simulink model "Fig221"  (R2014b)
settings: Solver=ode3  StartTime=0.0  StopTime=10.007  FixedStep=2e-5  RelTol=1e-5
undefined symbols (not defined in the file): gcbh, rcfiltgaincompat
libraries: commchan3 x1, commsink2 x1, dsparch4 x1, dspsigops x1, commrandsrc2 x1, commfilt2 x1
settings Model: Creator=Dennis Silage  LastModifiedBy=Silage
settings DataIOCC: SignalLoggingSaveFormat=ModelDataLogs
settings OptimizationCC: ExpressionDepthLimit=2147483647  InitFltsAndDblsToZero=on
settings DebuggingCC: UnderspecifiedInitializationDetection=Classic  MergeDetectMultiDrivingBlocksExec=none  SolverPrmCheckMsg=none  FcnCallInpInsideContextMsg=UseLocalSettings  StateNameClashWarn=warning
settings GRTTargetCC: CombineOutputUpdateFcns=off  GRTInterface=on

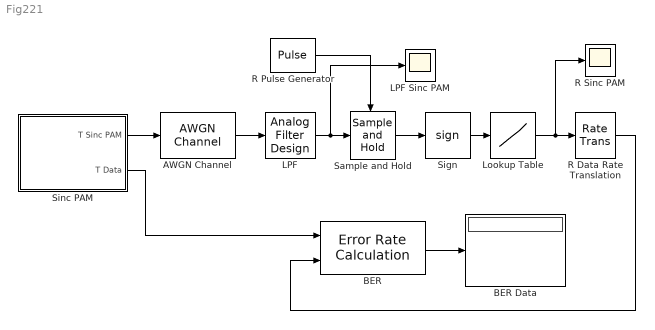
== system Fig221 ==
  AWGN Channel : commchan3/AWGN Channel  InputProcessing=Inherited (this choice will be removed - see release notes)  seed=randseed  noiseMode=Variance from mask  EbNodB=10  EsNodB=10  SNRdB=10  bitsPerSym=1  Ps=1  Tsym=1  variance=0
  BER : commsink2/Error Rate Calculation  N=8  st_delay=0  cp_mode=Entire frame  subframe=[]  PMode=Port  WsName=ErrorVec  RsMode2=off  stop=off  numErr=100  maxBits=1e6
  BER Data : Display
  LPF : dsparch4/Analog Filter Design  method=Chebyshev I  filttype=Lowpass  N=9  Wlo=2*pi*600  Whi=80  Rp=0.1  Rs=40
  LPF Sinc PAM : Scope
      settings: TimeRange=0.05  YMin=-8  YMax=8  SaveName=ScopeData3
  Lookup Table : Lookup_n-D  NumberOfTableDimensions=1  BreakpointsForDimension1=[-1,0,1]  BreakpointsForDimension3=[5, 7]  Table=[-1,-1,1]  InternalRulePriority=Speed  RndMeth=Simplest  InputSameDT=on
  R Data Rate Translation : RateTransition  OutPortSampleTime=1e-3
  R Pulse Generator : DiscretePulseGenerator  PulseType=Time based  Period=1e-3  PulseWidth=10
  R Sinc PAM : Scope
      settings: TimeRange=0.05  YMin=-8  YMax=8
  Sample and Hold : dspsigops/Sample and Hold  trig=Rising edge  initCond=0  latchinput=off
  Sign : Signum
  Sinc PAM : Subsystem
  wires:
  BER/1 -> BER Data/1
  R Pulse Generator/1 -> Sample and Hold/Trigger
  Sign/1 -> Lookup Table/1
  Sample and Hold/1 -> Sign/1
  Lookup Table/1 -> R Data Rate Translation/1, R Sinc PAM/1
  R Data Rate Translation/1 -> BER/2
  AWGN Channel/1 -> LPF/1
  LPF/1 -> Sample and Hold/1, LPF Sinc PAM/1
  Sinc PAM/1("T Sinc PAM ") -> AWGN Channel/1
  Sinc PAM/2(T Data) -> BER/1

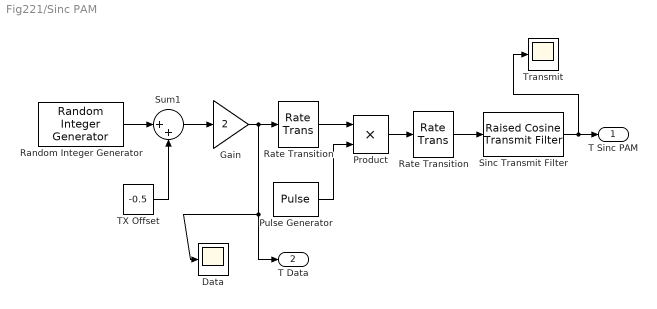
== system Fig221/Sinc PAM ==
  " Rate Transition" : RateTransition  OutPortSampleTime=1e-3
  Data : Scope
      settings: TimeRange=0.05  YMin=-8  YMax=8  SaveName=ScopeData2
  Gain : Gain  Gain=2
  Product : Product  RndMeth=Zero
  Pulse Generator : DiscretePulseGenerator  PulseType=Time based  Period=1e-3  PulseWidth=2
  Random Integer Generator : commrandsrc2/Random Integer Generator  mul=2  seed=randseed  Ts=1e-3  frameBased=off  sampPerFrame=50  orient=off  outDataType=double
  Rate Transition : RateTransition  OutPortSampleTime=2e-5
  Sinc Transmit Filter : commfilt2/Raised Cosine Transmit Filter  filtType=Normal  filtSpan=2*(4)  currentFiltSpan=2*(4)  D=4  R=0  sampMode=Mute  saveAsFlag=0  N=50  framing=Maintain input frame size  InputProcessing=Inherited (this choice will be removed - see release notes)  checkGain=User-specified  filterGain=(5)*rcfiltgaincompat(gcbh)  checkCoeff=off  variableName=rcTxFilt  launchFVT=off  roundingMode=Floor  overflowMode=off
  Sum1 : Sum  Inputs=|++
  TX Offset : Constant  Value=-0.5
  Transmit : Scope
      settings: TimeRange=0.05  YMin=-8  YMax=8
  "T Sinc PAM " : Outport
  T Data : Outport  Port=2
  wires:
  Sum1/1 -> Gain/1
  TX Offset/1 -> Sum1/2
  Random Integer Generator/1 -> Sum1/1
  Gain/1 -> Rate Transition/1, Data/1, T Data/1
  Rate Transition/1 -> Product/1
  Pulse Generator/1 -> Product/2
  " Rate Transition"/1 -> Sinc Transmit Filter/1
  Product/1 -> " Rate Transition"/1
  Sinc Transmit Filter/1 -> Transmit/1, "T Sinc PAM "/1
